simulink model "NI"  (R2017b)
settings: Solver=VariableStepAuto  StartTime=0.0  StopTime=40  RelTol=1e-3
libraries: Solver_SF x1, simulink x1
settings Model: Creator=lancer  LastModifiedBy=lancer

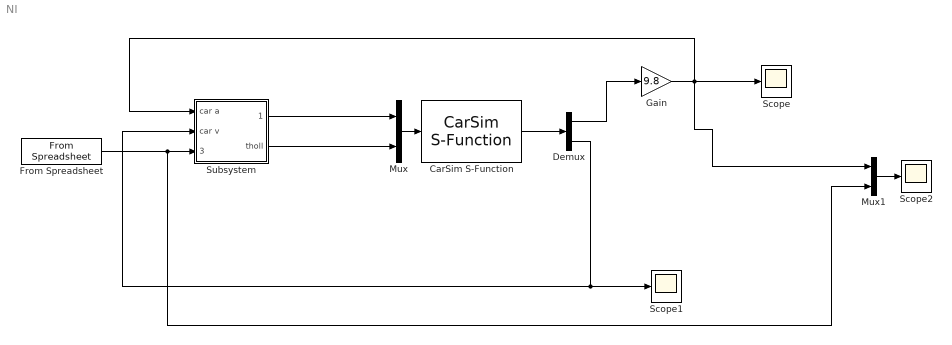
== system NI ==
  CarSim S-Function : Solver_SF/CarSim S-Function  Priority=1  VehicleCode=i_i  SIMFILE=simfile
  Demux : Demux  Outputs=2
  From Spreadsheet : FromSpreadsheet  FileName=C:\Users\lancer\Desktop\毕设\逆动力学模型\test.xlsx
  Gain : Gain  Gain=9.8
  Mux : Mux  Inputs=2
  Mux1 : Mux  Inputs=2
  Scope : Scope
  Scope1 : Scope
  Scope2 : Scope
  Subsystem : Subsystem
  wires:
  Mux/1 -> CarSim S-Function/1
  CarSim S-Function/1 -> Demux/1
  Demux/1 -> Gain/1
  Gain/1 -> Mux1/1, Subsystem/1(car a), Scope/1
  From Spreadsheet/1 -> Mux1/2, Subsystem/3(desire a)
  Mux1/1 -> Scope2/1
  Demux/2 -> Scope1/1, Subsystem/2(car v)
  Subsystem/1(brake1) -> Mux/1
  Subsystem/2(tholl) -> Mux/2

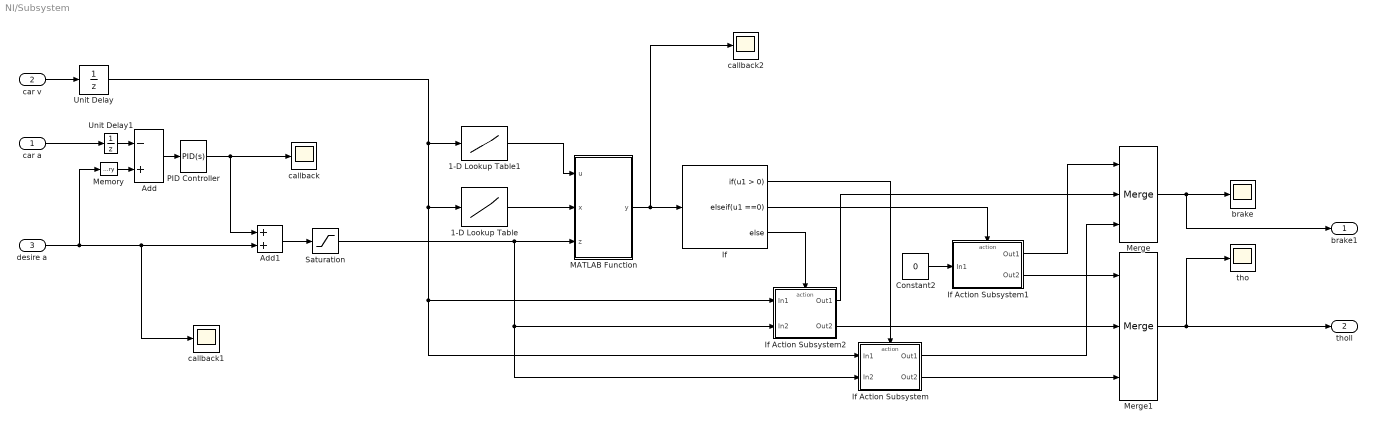
== system NI/Subsystem ==
  car a : Inport
  car v : Inport  Port=2
  desire a : Inport  Port=3
  1-D Lookup Table : Lookup_n-D  NumberOfTableDimensions=1  BreakpointsForDimension1=xlsread('tho0brk0','sheet2','A2:A29')  Table=xlsread('tho0brk0','sheet2','B2:B29')  InternalRulePriority=Speed  RndMeth=Simplest  InputSameDT=on
  1-D Lookup Table1 : Lookup_n-D  NumberOfTableDimensions=1  BreakpointsForDimension1=xlsread('tho0brk0','sheet3','A2:A29')  Table=xlsread('tho0brk0','sheet3','B2:B29')  InternalRulePriority=Speed  RndMeth=Simplest  InputSameDT=on
  Add : Sum  Inputs=-+
  Add1 : Sum
  Constant2 : Constant  Value=0
  If : If  ElseIfExpressions=u1 ==0
  If Action Subsystem : Subsystem  TreatAsAtomicUnit=on
  If Action Subsystem1 : Subsystem  TreatAsAtomicUnit=on
  If Action Subsystem2 : Subsystem  TreatAsAtomicUnit=on
  MATLAB Function : MATLAB Function  TreatAsAtomicUnit=on
  Memory : Memory
  Merge : Merge  Inputs=3
  Merge1 : Merge  Inputs=3
  PID Controller : simulink/Continuous/PID Controller  Controller=PID  TimeDomain=Continuous-time  SampleTime=-1  IntegratorMethod=Forward Euler  FilterMethod=Forward Euler  Form=Parallel  UseFilter=on  ControllerParametersSource=internal  P=2.2  I=0  D=0  N=100  InitialConditionSource=internal  InitialConditionForIntegrator=0  InitialConditionForFilter=0  ExternalReset=none  LimitOutput=off  UpperSaturationLimit=inf  LowerSaturationLimit=-inf  LinearizeAsGain=on  AntiWindupMode=none  Kb=1  TrackingMode=off  Kt=1  PParamMin=[]  PParamMax=[]  IParamMin=[]  IParamMax=[]  DParamMin=[]  DParamMax=[]  NParamMin=[]  NParamMax=[]  KbParamMin=[]  KbParamMax=[]  KtParamMin=[]  KtParamMax=[]  POutMin=[]  POutMax=[]  IOutMin=[]  IOutMax=[]  DOutMin=[]  DOutMax=[]  NOutMin=[]  NOutMax=[]  KbOutMin=[]  KbOutMax=[]  KtOutMin=[]  KtOutMax=[]  IntegratorOutMin=[]  IntegratorOutMax=[]  FilterOutMin=[]  FilterOutMax=[]  SumOutMin=[]  SumOutMax=[]  SumI1OutMin=[]  SumI1OutMax=[]  SumI2OutMin=[]  SumI2OutMax=[]  SumI3OutMin=[]  SumI3OutMax=[]  SumDOutMin=[]  SumDOutMax=[]  SaturationOutMin=[]  SaturationOutMax=[]  IntegratorContinuousStateAttributes=''  IntegratorStateMustResolveToSignalObject=off  IntegratorRTWStateStorageClass=Auto  FilterContinuousStateAttributes=''  FilterStateMustResolveToSignalObject=off  FilterRTWStateStorageClass=Auto  DifferentiatorICPrevScaledInput=0  DifferentiatorOutMin=[]  DifferentiatorOutMax=[]  InitialConditionSetting=State (most efficient)  FilterDiffOutCoefMin=[]  FilterDiffOutCoefMax=[]  SumDenOutMin=[]  SumDenOutMax=[]  SumNumOutMin=[]  SumNumOutMax=[]  ReciprocalOutMin=[]  ReciprocalOutMax=[]  DivideOutMin=[]  DivideOutMax=[]  TunerSelectOption=Transfer Function Based (PID Tuner App)
  Saturation : Saturate  UpperLimit=5.4  LowerLimit=-5
  Unit Delay : UnitDelay  SampleTime=-1
  Unit Delay1 : UnitDelay  SampleTime=-1
  brake : Scope
  callback : Scope
  callback1 : Scope
  callback2 : Scope
  tho : Scope
  brake1 : Outport
  tholl : Outport  Port=2
  wires:
  car v/1 -> Unit Delay/1
  car a/1 -> Unit Delay1/1
  desire a/1 -> callback1/1, Add1/2, Memory/1
  If Action Subsystem1/2(Out2) -> Merge1/1
  Add1/1 -> Saturation/1
  PID Controller/1 -> Add1/1, callback/1
  1-D Lookup Table1/1 -> MATLAB Function/1(u)
  If Action Subsystem2/1(Out1) -> Merge/2
  Constant2/1 -> If Action Subsystem1/1(In1)
  If Action Subsystem1/1(Out1) -> Merge/1
  If/2 -> If Action Subsystem1/Action
  Saturation/1 -> If Action Subsystem/2(In2), If Action Subsystem2/2(In2), MATLAB Function/3(z)
  If/1 -> If Action Subsystem/Action
  MATLAB Function/1(y) -> callback2/1, If/1
  If Action Subsystem/1(Out1) -> Merge/3
  If Action Subsystem/2(Out2) -> Merge1/3
  Merge/1 -> brake1/1, brake/1
  If Action Subsystem2/2(Out2) -> Merge1/2
  Merge1/1 -> tholl/1, tho/1
  If/3 -> If Action Subsystem2/Action
  Unit Delay/1 -> 1-D Lookup Table1/1, If Action Subsystem/1(In1), If Action Subsystem2/1(In1), 1-D Lookup Table/1
  Memory/1 -> Add/2
  1-D Lookup Table/1 -> MATLAB Function/2(x)
  Add/1 -> PID Controller/1
  Unit Delay1/1 -> Add/1

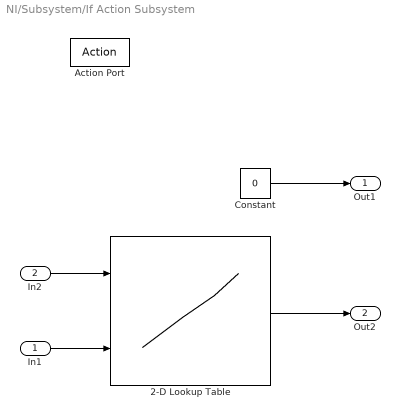
== system NI/Subsystem/If Action Subsystem ==
  In1 : Inport
  In2 : Inport  Port=2
  Action Port : ActionPort  ActionType=then
  2-D Lookup Table : Lookup_n-D  BreakpointsForDimension1=xlsread('tho-v-a','sheet4','A3:A34')  BreakpointsForDimension2=xlsread('tho-v-a','sheet4','B2:P2')  Table=xlsread('tho-v-a','sheet4','B3:P34')  InternalRulePriority=Speed  RndMeth=Simplest  InputSameDT=on
  Constant : Constant  Value=0
  Out1 : Outport
  Out2 : Outport  Port=2
  wires:
  Constant/1 -> Out1/1
  2-D Lookup Table/1 -> Out2/1
  In2/1 -> 2-D Lookup Table/1
  In1/1 -> 2-D Lookup Table/2

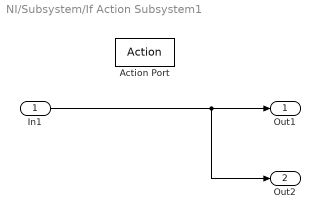
== system NI/Subsystem/If Action Subsystem1 ==
  In1 : Inport
  Action Port : ActionPort  ActionType=elseif
  Out1 : Outport
  Out2 : Outport  Port=2
  wires:
  In1/1 -> Out2/1, Out1/1

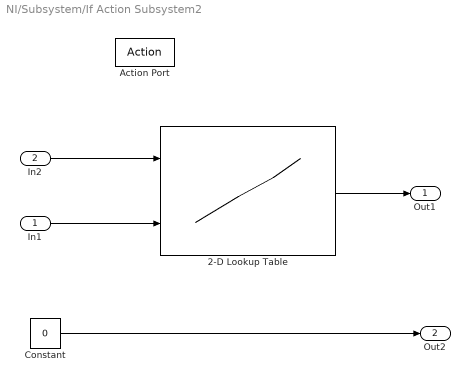
== system NI/Subsystem/If Action Subsystem2 ==
  In1 : Inport
  In2 : Inport  Port=2
  Action Port : ActionPort  ActionType=else
  2-D Lookup Table : Lookup_n-D  BreakpointsForDimension1=xlsread('brk-v-a','sheet3','A3:A28')  BreakpointsForDimension2=xlsread('brk-v-a','sheet3','B2:P2')  Table=xlsread('brk-v-a','sheet3','B3:P28')  InternalRulePriority=Speed  RndMeth=Simplest  InputSameDT=on
  Constant : Constant  Value=0
  Out1 : Outport
  Out2 : Outport  Port=2
  wires:
  2-D Lookup Table/1 -> Out1/1
  Constant/1 -> Out2/1
  In2/1 -> 2-D Lookup Table/1
  In1/1 -> 2-D Lookup Table/2

== matlab function NI/Subsystem/MATLAB Function ==
  data: u input; y output; x input; z input
function y = fcn(u, x, z)
if z>u
    y=1;
elseif z<u&&z>x
    y=0;
elseif z<x
    y=-1;
else
    y=5;
end
